simulink model "AttitudeControl_ADRC_FLY"  (R2017b)
settings: Solver=FixedStepDiscrete  StartTime=0.0  StopTime=10.0  RelTol=1e-3
undefined symbols (not defined in the file): DiscIntNeverNeededParam, Kd_YAW_AngleRate, Ki_YAW_AngleRate, Kp_YAW_AngleRate, RC1_MAX, RC1_MIN, RC2_MAX, RC2_MIN, RC3_MAX, RC3_MIN, RC4_MAX, RC4_MIN, RGBLED_COLOR_ENUM, RGBLED_MODE_ENUM, Saturation_I_Y_Max, Saturation_I_Y_Min, SL_ESO_B0, SL_ESO_B01, SL_ESO_B02, SL_ESO_B03, SL_ESO_D, SL_ESO_H, SL_NLSEF_C, SL_NLSEF_H, SL_NLSEF_R, SL_TD_H, SL_TD_R, tau2sigma, THR_HOVER
libraries: pixhawk_slib_sensors_actuators x5, simulink x2, pixhawk_slib_misc_utils x2
settings Model: Creator=wsh  LastModifiedBy=Mr Wang
settings OptimizationCC: DefaultParameterBehavior=Inlined  MaxStackSize=64
settings DebuggingCC: ParameterTunabilityLossMsg=error
settings HardwareCC: ProdBitPerPointer=32  ProdBitPerSizeT=32  ProdBitPerPtrDiffT=32  ProdLargestAtomicInteger=Long  ProdLargestAtomicFloat=Double  ProdWordSize=32  ProdHWDeviceType=ARM Compatible->ARM Cortex
settings SFSimCC: MATLABDynamicMemAlloc=off
settings RTWCC: SystemTargetFile=ert.tlc  HardwareBoard=Pixhawk PX4  TemplateMakefile=ert_default_tmf  GenerateReport=on  CustomSource=px4_simulink_app_params.c  Toolchain=Pixhawk Toolchain  IncludeHyperlinkInReport=on  LaunchReport=on  GenerateTraceInfo=on  GenerateTraceReport=on  GenerateTraceReportSl=on  GenerateTraceReportSf=on  GenerateTraceReportEml=on
settings CodeAppCC: ForceParamTrailComments=on  IgnoreCustomStorageClasses=off  OperatorAnnotations=on  SimulinkDataObjDesc=on  SFDataObjDesc=on  MATLABFcnDesc=on  InsertBlockDesc=on  StateflowObjectComments=on  MATLABSourceComments=on
settings ERTTargetCC: MultiwordLength=2048  ERTCustomFileTemplate=PX4_codertarget_file_process.tlc

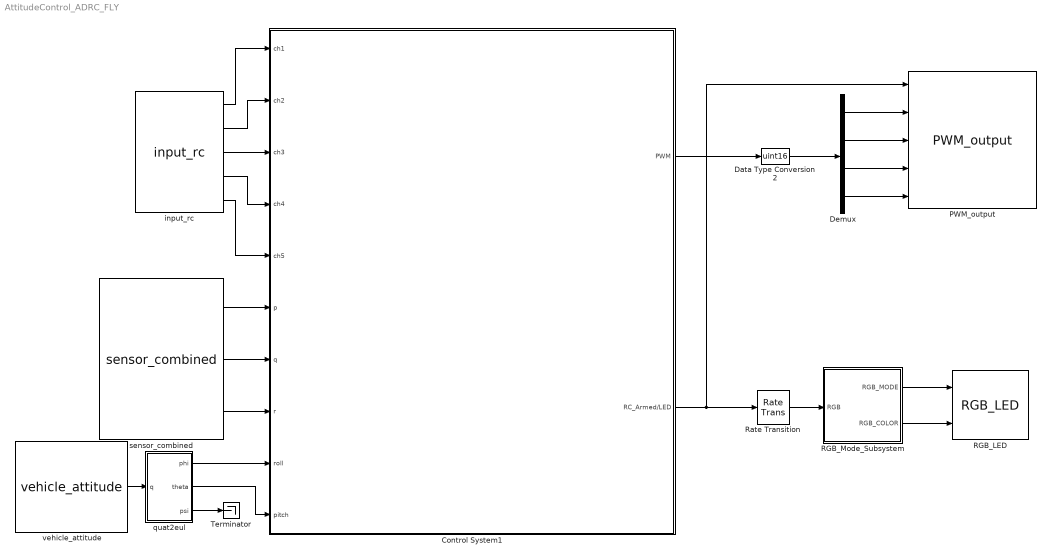
== system AttitudeControl_ADRC_FLY ==
  Control System1 : Subsystem
      mask Display: image('icon\pixhawk.png');
  Data Type Conversion2 : DataTypeConversion  OutDataTypeStr=uint16
  Demux : Demux
  PWM_output : pixhawk_slib_sensors_actuators/PWM_output  Description=|  pub_outputs=on  pwm_rate=400Hz  show_pwm1=on  show_pwm5=off  show_pwm2=on  show_pwm6=off  show_pwm3=on  show_pwm7=off  show_pwm4=on  show_pwm8=off
      | This block allows the user to send the appropriate PWM signals out to the PX4 outputs.  
      | These are usually connected to the ESCs which control the motor speeds. 
      | In order for the flight control to arm (enable) the output from the software side, the ARM Output input must be held high (boolean TRUE).  
      | Only then will the PWM values be sent out the PX4 hardware ports.  
      | This is usually a function of the RC Tx in combination with other flight modes programmed in the Simulink model by the user.  
      | The block has 8 available ports (data type uint16) which can be selectively chosen.  
      | These correspond to the 8 PWM output ports on the px4fmu hardware.
      settings: SourceProductName=Pixhawk Target Blocks
  RGB_LED : pixhawk_slib_sensors_actuators/RGB_LED
      settings: SourceProductName=Pixhawk Target Blocks
  RGB_Mode_Subsystem : Subsystem
  Rate Transition : RateTransition  OutPortSampleTime=1
  Terminator : Terminator
  input_rc : pixhawk_slib_sensors_actuators/input_rc  Description=|  sampletime=0.004  channel1=on  channel2=on  channel3=on  channel4=on  channel5=on  channel6=off  channel7=off  channel8=off  channel9=off  channel10=off  channel11=off  channel12=off  channel13=off  channel14=off  channel15=off  channel16=off  channel17=off  channel18=off  ch_count=off  rssi=off  rc_failsafe=off  rc_lost=off  rc_inputsource=off
      | RC Input Block
      | 
      | This block provides user input control to the model.
      | It uses the input_rc uORB topic.
      | 
      | The user has the ability to choose which channels are available as outputs from this block and also some optional outputs. These include 
      | Channels 1 through 18
      | double data type indicating the PWM value from the controller 
      | measured pulse widths for each of the supported channels 
      | Channel Count 
      | uint32 data type of the number of channels which are detector by the PX4 
      | RC Failsafe 
      | boolean data types indicating that the RC Tx is sending the FailSafe signal (if equipped and properly setup) 
      | explicit failsafe flag: true on TX failure or TX out of range , false otherwise. 
      | Only the true state is reliable, as there are some (PPM) receivers on the market going into failsafe without telling us explicitly. 
      | RC Input Source 
      | Enumeration data type indicating which source the RC input is from. 
      | Valid values are found in the ENUM file: RC_INPUT_SOURCE_ENUM.m 
      |           Enumeration members for class 'RC_INPUT_SOURCE_ENUM':
      |           RCINPUT_SOURCE_UNKNOWN         (0)
      |           RCINPUT_SOURCE_PX4FMU_PPM      (1)
      |           RCINPUT_SOURCE_PX4IO_PPM       (2)
      |           RCINPUT_SOURCE_PX4IO_SPEKTRUM  (3)
      |           RCINPUT_SOURCE_PX4IO_SBUS      (4)
      |           RCINPUT_SOURCE_PX4IO_ST24      (5)
      |           RCINPUT_SOURCE_MAVLINK         (6)
      |           RCINPUT_SOURCE_QURT            (7)
      |           RCINPUT_SOURCE_PX4FMU_SPEKTRUM (8)
      |           RCINPUT_SOURCE_PX4FMU_SBUS     (9)
      |           RCINPUT_SOURCE_PX4FMU_ST24     (10)
      |           RCINPUT_SOURCE_PX4FMU_SUMD     (11)
      |           RCINPUT_SOURCE_PX4FMU_DSM      (12)
      |           RCINPUT_SOURCE_PX4IO_SUMD      (13)
      | 
      | RSSI - Receive signal strength index 
      | receive signal strength indicator (RSSI): < 0: Undefined, 0: no signal, 255: full reception 
      | RC Lost Connection 
      | boolean data type indicating RC receiver connection status 
      | True, if no frame has arrived in the expected time, false otherwise. 
      | True usally means that the receiver has been disconnected, but can also indicate a radio link loss on "stupid" systems. 
      | Will remain false, if a RX with failsafe option continues to transmit frames after a link loss. 
      |   
      | Sample Model: px4demo_input_rc.slx
      settings: SourceProductName=Pixhawk Target Blocks
  quat2eul : MATLAB Function  TreatAsAtomicUnit=on
  sensor_combined : pixhawk_slib_sensors_actuators/sensor_combined  Description=|  sampletime=0.004  show_mag=off  show_acc=off  show_gyro=on  show_baro=off  show_ts=off
      | Sensor Combined Block
      | 
      | This block enables access to the various sensors available on the px4fmu-v2 hardware.  
      | The user can use these signals in the Simulink control model.  
      | The sample time needs to be provided in the mask dialog.  
      | Optional output ports can also be selected.  
      | Refer to the sample model: px4demo_attitude_control.slx
      | 
      | Signal definitions: 
      | Magnetometer (x,y,z) - single values – Magnetic field in NED body frame, in Gauss 
      | Accelerometer (x,y,z) - single values – Acceleration in NED body frame, in m/s^2 
      | Gyroscope (p,q,r) - single values – Angular velocity in radians per second 
      | Barometer (Altitude) - single value – Barometric pressure, already temperature compensated (millibars) 
      | RunTime (timestamp) - double value – Timestamp in microseconds since boot, from gyro 
      |   
      | The sensor_combined block needs to have the px4io service running on the PX4 hardware in order to get valid signal values.
      settings: SourceProductName=Pixhawk Target Blocks
  vehicle_attitude : pixhawk_slib_sensors_actuators/vehicle_attitude  Description=|  sampletime=0.004  show_r=off  show_p=off  show_y=off  show_q=on  show_ts=off
      | This block gives access to the running service that calculates the vehicle’s attitude.  A uORB topic (vehicle_attitude (attitude measurements)) publisher MUST be running in order for this block to provide valid signal values.  The available ones as of v1.3 are: 
      | attitude_estimator_ekf – EKF-Extended Kalman Filter for attitude estimation 
      | attitude_estimator_so3 – SO(3)-attitude estimation by using accelerometer, gyroscopes and magnetometer 
      | One of these MUST be running on the px4fmu in order for this block to return valid values.  Refer to the sample model: px4demo_attitude_control.slx. Attitude in NED (North-East-Down) body frame in SI units. 
      | Signal definitions: 
      | Roll – single value, Roll angle (rad, Tait-Bryan, NED) 
      | Pitch – single value, Pitch angle (rad, Tait-Bryan, NED) 
      | Yaw – single value, Yaw angle (rad, Tait-Bryan, NED) 
      | Quaternion (NED) – single(4) values (optional based on the uORB publisher)
      settings: SourceProductName=Pixhawk Target Blocks
  wires:
  sensor_combined/1 -> Control System1/6(p)
  sensor_combined/3 -> Control System1/8(r)
  sensor_combined/2 -> Control System1/7(q)
  input_rc/1 -> Control System1/1(ch1)
  input_rc/2 -> Control System1/2(ch2)
  input_rc/3 -> Control System1/3(ch3)
  input_rc/4 -> Control System1/4(ch4)
  input_rc/5 -> Control System1/5(ch5)
  quat2eul/2(theta) -> Control System1/10(pitch)
  quat2eul/3(psi) -> Terminator/1
  quat2eul/1(phi) -> Control System1/9(roll)
  vehicle_attitude/1 -> quat2eul/1(q)
  RGB_Mode_Subsystem/1(RGB_MODE) -> RGB_LED/1
  Rate Transition/1 -> RGB_Mode_Subsystem/1(RGB)
  RGB_Mode_Subsystem/2(RGB_COLOR) -> RGB_LED/2
  Control System1/2(RC_Armed/LED) -> PWM_output/1, Rate Transition/1
  Demux/3 -> PWM_output/4
  Data Type Conversion2/1 -> Demux/1
  Control System1/1(PWM) -> Data Type Conversion2/1
  Demux/4 -> PWM_output/5
  Demux/1 -> PWM_output/2
  Demux/2 -> PWM_output/3

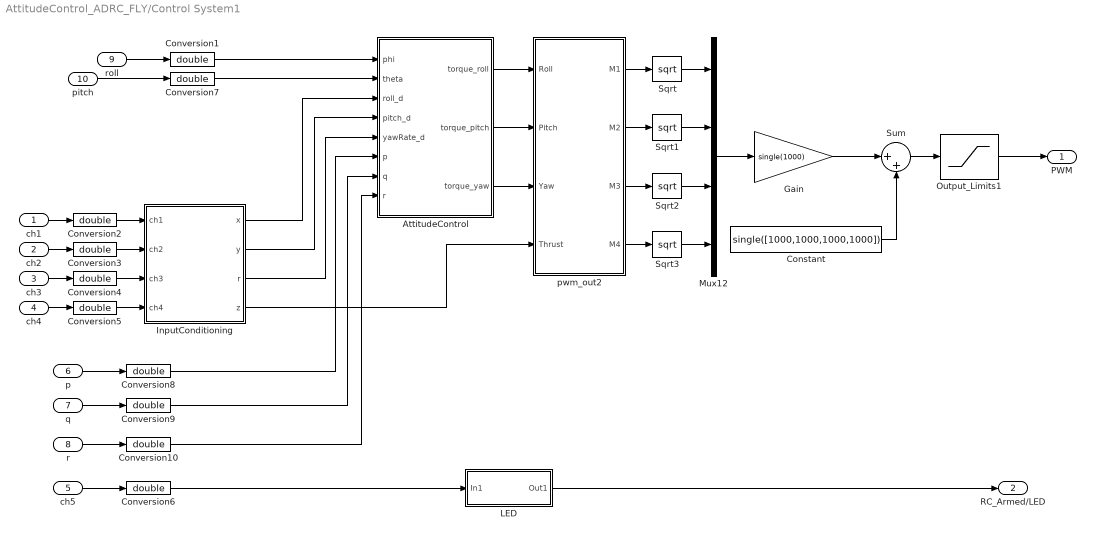
== system AttitudeControl_ADRC_FLY/Control System1 ==
  ch1 : Inport  OutDataTypeStr=uint16  PortDimensions=1
  ch2 : Inport  Port=2  OutDataTypeStr=uint16  PortDimensions=1
  ch3 : Inport  Port=3  OutDataTypeStr=uint16  PortDimensions=1
  ch4 : Inport  Port=4  OutDataTypeStr=uint16  PortDimensions=1
  ch5 : Inport  Port=5  OutDataTypeStr=uint16  PortDimensions=1  Interpolate=off
  p : Inport  Port=6  PortDimensions=1
  q : Inport  Port=7  PortDimensions=1
  r : Inport  Port=8  PortDimensions=1
  roll : Inport  Port=9  PortDimensions=1
  pitch : Inport  Port=10  PortDimensions=1
  AttitudeControl : Subsystem
  Constant : Constant  Value=single([1000,1000,1000,1000])
  Conversion{1..10} (10 alike) : DataTypeConversion  OutDataTypeStr=double
  Gain : Gain  Gain=single(1000)
  InputConditioning : Subsystem
  "LED " : Subsystem
  Mux12 : Mux
  Output_Limits1 : Saturate  Priority=2  UpperLimit=2000  LowerLimit=1000
  Sqrt{,1..3} (4 alike) : Sqrt  SaturateOnIntegerOverflow=on
  Sum : Sum  Inputs=|++
  pwm_out2 : MATLAB Function  SystemSampleTime=0.004
  PWM : Outport
  RC_Armed/LED : Outport  Port=2  PortDimensions=1
  wires:
  ch3/1 -> Conversion4/1
  ch5/1 -> Conversion6/1
  r/1 -> Conversion10/1
  q/1 -> Conversion9/1
  InputConditioning/3(r) -> AttitudeControl/5(yawRate_d)
  p/1 -> Conversion8/1
  ch4/1 -> Conversion5/1
  "LED "/1(Out1) -> RC_Armed/LED/1
  Conversion6/1 -> "LED "/1(In1)
  Conversion5/1 -> InputConditioning/4(ch4)
  Conversion4/1 -> InputConditioning/3(ch3)
  pitch/1 -> Conversion7/1
  roll/1 -> Conversion1/1
  ch1/1 -> Conversion2/1
  ch2/1 -> Conversion3/1
  Conversion1/1 -> AttitudeControl/1(phi)
  Conversion7/1 -> AttitudeControl/2(theta)
  Conversion8/1 -> AttitudeControl/6(p)
  Conversion9/1 -> AttitudeControl/7(q)
  Conversion10/1 -> AttitudeControl/8(r)
  Conversion2/1 -> InputConditioning/1("ch1 ")
  Conversion3/1 -> InputConditioning/2(ch2)
  InputConditioning/1(x) -> AttitudeControl/3(roll_d)
  InputConditioning/2(y) -> AttitudeControl/4(pitch_d)
  Constant/1 -> Sum/2
  Gain/1 -> Sum/1
  Mux12/1 -> Gain/1
  Sqrt3/1 -> Mux12/4
  Sqrt1/1 -> Mux12/2
  Sqrt/1 -> Mux12/1
  InputConditioning/4(z) -> pwm_out2/4(Thrust)
  pwm_out2/1(M1) -> Sqrt/1
  pwm_out2/2(M2) -> Sqrt1/1
  AttitudeControl/2(torque_pitch) -> pwm_out2/2(Pitch)
  AttitudeControl/1(torque_roll) -> pwm_out2/1(Roll)
  Sum/1 -> Output_Limits1/1
  Sqrt2/1 -> Mux12/3
  AttitudeControl/3(torque_yaw) -> pwm_out2/3(Yaw)
  pwm_out2/3(M3) -> Sqrt2/1
  pwm_out2/4(M4) -> Sqrt3/1
  Output_Limits1/1 -> PWM/1

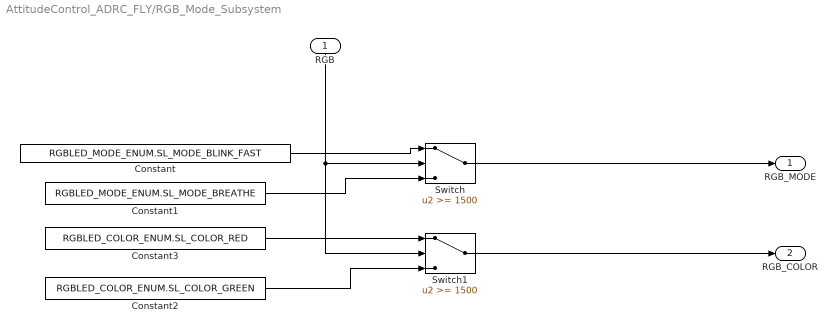
== system AttitudeControl_ADRC_FLY/RGB_Mode_Subsystem ==
  RGB : Inport
  Constant : Constant  Value=RGBLED_MODE_ENUM.SL_MODE_BLINK_FAST  OutDataTypeStr=Enum: RGBLED_MODE_ENUM
  Constant1 : Constant  Value=RGBLED_MODE_ENUM.SL_MODE_BREATHE  OutDataTypeStr=Enum: RGBLED_MODE_ENUM
  Constant2 : Constant  Value=RGBLED_COLOR_ENUM.SL_COLOR_GREEN  OutDataTypeStr=Enum: RGBLED_COLOR_ENUM
  Constant3 : Constant  Value=RGBLED_COLOR_ENUM.SL_COLOR_RED  OutDataTypeStr=Enum: RGBLED_COLOR_ENUM
  Switch : Switch  Threshold=1500
  Switch1 : Switch  Threshold=1500
  RGB_MODE : Outport
  RGB_COLOR : Outport  Port=2
  wires:
  Switch1/1 -> RGB_COLOR/1
  Constant2/1 -> Switch1/3
  Constant3/1 -> Switch1/1
  Switch/1 -> RGB_MODE/1
  Constant1/1 -> Switch/3
  Constant/1 -> Switch/1
  RGB/1 -> Switch/2, Switch1/2

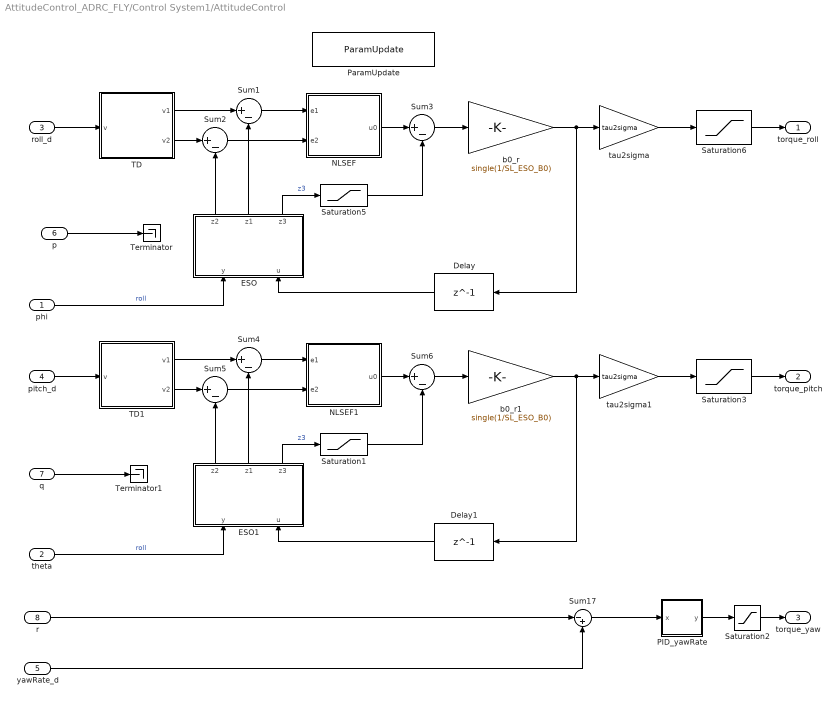
== system AttitudeControl_ADRC_FLY/Control System1/AttitudeControl ==
  phi : Inport
  theta : Inport  Port=2
  roll_d : Inport  Port=3
  pitch_d : Inport  Port=4
  yawRate_d : Inport  Port=5
  p : Inport  Port=6
  q : Inport  Port=7
  r : Inport  Port=8
  Delay : Delay  DelayLength=1  InitialCondition=0
  Delay1 : Delay  DelayLength=1  InitialCondition=0
  ESO : Subsystem
  ESO1 : Subsystem
  NLSEF : Subsystem
  NLSEF1 : Subsystem
  PID_yawRate : Subsystem
  ParamUpdate : pixhawk_slib_misc_utils/ParamUpdate  Description=|  Unformatted_StrSet=0  TLC_StrSet=0  NumParams=0  Ts=0
      | ParamUpdate Block
      | 
      | Use this block at your top-level of your model to insert a "parameter update" function in the generated code.
      settings: SourceProductName=Pixhawk Target Blocks
  Saturation1 : Saturate  UpperLimit=SL_NLSEF_R*0.5  LowerLimit=-SL_NLSEF_R*0.5
  Saturation2 : Saturate
  Saturation3 : Saturate  UpperLimit=0.4  LowerLimit=-0.4
  Saturation5 : Saturate  UpperLimit=SL_NLSEF_R*0.5  LowerLimit=-SL_NLSEF_R*0.5
  Saturation6 : Saturate  UpperLimit=0.4  LowerLimit=-0.4
  Sum{1..6} (6 alike) : Sum  Inputs=|+-
  Sum17 : Sum  Inputs=|-+
  TD : Subsystem
  TD1 : Subsystem
  Terminator : Terminator
  Terminator1 : Terminator
  b0_r : Gain  Gain=single(1/SL_ESO_B0)
  b0_r1 : Gain  Gain=single(1/SL_ESO_B0)
  tau2sigma : Gain  Gain=tau2sigma
  tau2sigma1 : Gain  Gain=tau2sigma
  torque_roll : Outport
  torque_pitch : Outport  Port=2
  torque_yaw : Outport  Port=3
  wires:
  r/1 -> Sum17/1
  Sum17/1 -> PID_yawRate/1(x)
  PID_yawRate/1(y) -> Saturation2/1
  yawRate_d/1 -> Sum17/2
  Saturation2/1 -> torque_yaw/1
  ESO/1(z2) -> Sum2/2
  ESO/3(z3) -> Saturation5/1  "z3"
  roll_d/1 -> TD/1(v)
  ESO/2(z1) -> Sum1/2
  Saturation5/1 -> Sum3/2
  Sum3/1 -> b0_r/1
  TD/1(v1) -> Sum1/1
  Delay/1 -> ESO/2(u)
  tau2sigma/1 -> Saturation6/1
  b0_r/1 -> tau2sigma/1, Delay/1
  Sum1/1 -> NLSEF/1(e1)
  phi/1 -> ESO/1(y)  "roll"
  NLSEF/1(u0) -> Sum3/1
  Saturation6/1 -> torque_roll/1
  TD/2(v2) -> Sum2/1
  Sum2/1 -> NLSEF/2(e2)
  theta/1 -> ESO1/1(y)  "roll"
  pitch_d/1 -> TD1/1(v)
  Sum5/1 -> NLSEF1/2(e2)
  TD1/2(v2) -> Sum5/1
  NLSEF1/1(u0) -> Sum6/1
  Delay1/1 -> ESO1/2(u)
  Saturation3/1 -> torque_pitch/1
  b0_r1/1 -> tau2sigma1/1, Delay1/1
  TD1/1(v1) -> Sum4/1
  tau2sigma1/1 -> Saturation3/1
  Sum4/1 -> NLSEF1/1(e1)
  ESO1/3(z3) -> Saturation1/1  "z3"
  Saturation1/1 -> Sum6/2
  ESO1/2(z1) -> Sum4/2
  ESO1/1(z2) -> Sum5/2
  Sum6/1 -> b0_r1/1
  p/1 -> Terminator/1
  q/1 -> Terminator1/1

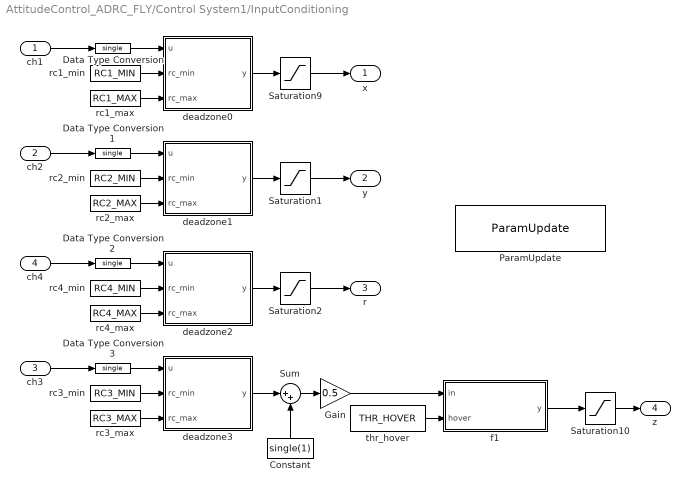
== system AttitudeControl_ADRC_FLY/Control System1/InputConditioning ==
  "ch1 " : Inport
  ch2 : Inport  Port=2
  ch3 : Inport  Port=3
  ch4 : Inport  Port=4
  Constant : Constant  Value=single(1)
  Data Type Conversion{,1..3} (4 alike) : DataTypeConversion  OutDataTypeStr=single
  Gain : Gain  Gain=0.5  ParamDataTypeStr=single  OutDataTypeStr=single
  ParamUpdate : pixhawk_slib_misc_utils/ParamUpdate  Description=|  Unformatted_StrSet=0  TLC_StrSet=0  NumParams=0  Ts=0
      | ParamUpdate Block
      | 
      | Use this block at your top-level of your model to insert a "parameter update" function in the generated code.
      settings: SourceProductName=Pixhawk Target Blocks
  Saturation1 : Saturate  UpperLimit=1  LowerLimit=-1
  Saturation10 : Saturate  UpperLimit=1  LowerLimit=0
  Saturation2 : Saturate  UpperLimit=1  LowerLimit=-1
  Saturation9 : Saturate  UpperLimit=1  LowerLimit=-1
  Sum : Sum  Inputs=|++
  deadzone0 : MATLAB Function  TreatAsAtomicUnit=on
  deadzone1 : MATLAB Function  TreatAsAtomicUnit=on
  deadzone2 : MATLAB Function  TreatAsAtomicUnit=on
  deadzone3 : MATLAB Function  TreatAsAtomicUnit=on
  f1 : MATLAB Function  TreatAsAtomicUnit=on
  rc1_max : Constant  Value=RC1_MAX
  rc1_min : Constant  Value=RC1_MIN
  rc2_max : Constant  Value=RC2_MAX
  rc2_min : Constant  Value=RC2_MIN
  rc3_max : Constant  Value=RC3_MAX
  rc3_min : Constant  Value=RC3_MIN
  rc4_max : Constant  Value=RC4_MAX
  rc4_min : Constant  Value=RC4_MIN
  "thr_hover " : Constant  Value=THR_HOVER  OutDataTypeStr=single
  x : Outport
  y : Outport  Port=2
  r : Outport  Port=3
  z : Outport  Port=4
  wires:
  f1/1(y) -> Saturation10/1
  Gain/1 -> f1/1(in)
  "thr_hover "/1 -> f1/2(hover)
  Sum/1 -> Gain/1
  Constant/1 -> Sum/2
  "ch1 "/1 -> Data Type Conversion/1
  deadzone0/1(y) -> Saturation9/1
  Saturation10/1 -> z/1
  deadzone3/1(y) -> Sum/1
  rc1_min/1 -> deadzone0/2(rc_min)
  rc1_max/1 -> deadzone0/3(rc_max)
  Data Type Conversion/1 -> deadzone0/1(u)
  Data Type Conversion1/1 -> deadzone1/1(u)
  rc2_max/1 -> deadzone1/3(rc_max)
  rc2_min/1 -> deadzone1/2(rc_min)
  deadzone1/1(y) -> Saturation1/1
  ch2/1 -> Data Type Conversion1/1
  Data Type Conversion2/1 -> deadzone2/1(u)
  rc4_max/1 -> deadzone2/3(rc_max)
  rc4_min/1 -> deadzone2/2(rc_min)
  deadzone2/1(y) -> Saturation2/1
  ch4/1 -> Data Type Conversion2/1
  Saturation2/1 -> r/1
  ch3/1 -> Data Type Conversion3/1
  rc3_min/1 -> deadzone3/2(rc_min)
  rc3_max/1 -> deadzone3/3(rc_max)
  Data Type Conversion3/1 -> deadzone3/1(u)
  Saturation9/1 -> x/1
  Saturation1/1 -> y/1

== system AttitudeControl_ADRC_FLY/Control System1/LED  ==
  In1 : Inport
  Compare To Constant3 : simulink/Logic and Bit Operations/Compare To Constant  relop=>=  const=uint16(1500)  OutDataTypeStr=boolean
  Out1 : Outport
  wires:
  Compare To Constant3/1 -> Out1/1
  In1/1 -> Compare To Constant3/1

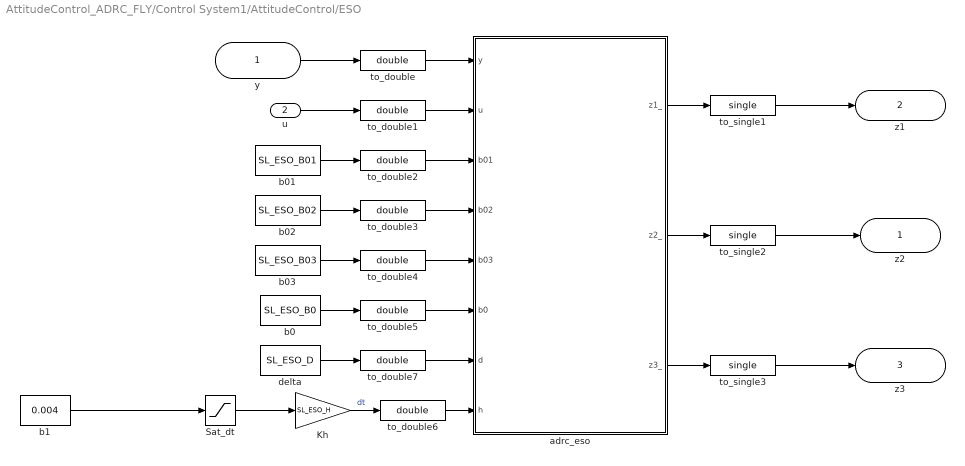
== system AttitudeControl_ADRC_FLY/Control System1/AttitudeControl/ESO ==
  y : Inport
  u : Inport  Port=2
  Kh : Gain  Priority=4  Gain=SL_ESO_H
  Sat_dt : Saturate  UpperLimit=0.02  LowerLimit=0.004
  adrc_eso : MATLAB Function  TreatAsAtomicUnit=on
  b0 : Constant  Value=SL_ESO_B0
  b01 : Constant  Value=SL_ESO_B01
  b02 : Constant  Value=SL_ESO_B02
  b03 : Constant  Value=SL_ESO_B03
  b1 : Constant  Value=0.004
  delta : Constant  Value=SL_ESO_D
  to_double{,1..7} (8 alike) : DataTypeConversion  OutDataTypeStr=double
  to_single1 : DataTypeConversion  OutDataTypeStr=single
  to_single2 : DataTypeConversion  OutDataTypeStr=single
  to_single3 : DataTypeConversion  OutDataTypeStr=single
  z2 : Outport
  z1 : Outport  Port=2  OutDataTypeStr=single
  z3 : Outport  Port=3
  wires:
  y/1 -> to_double/1
  u/1 -> to_double1/1
  b1/1 -> Sat_dt/1
  Sat_dt/1 -> Kh/1
  Kh/1 -> to_double6/1  "dt"
  adrc_eso/1(z1_) -> to_single1/1
  adrc_eso/2(z2_) -> to_single2/1
  adrc_eso/3(z3_) -> to_single3/1
  b01/1 -> to_double2/1
  b02/1 -> to_double3/1
  b03/1 -> to_double4/1
  b0/1 -> to_double5/1
  to_double/1 -> adrc_eso/1(y)
  to_double1/1 -> adrc_eso/2(u)
  to_double2/1 -> adrc_eso/3(b01)
  to_double3/1 -> adrc_eso/4(b02)
  to_double4/1 -> adrc_eso/5(b03)
  to_double5/1 -> adrc_eso/6(b0)
  to_single1/1 -> z1/1
  to_single2/1 -> z2/1
  to_single3/1 -> z3/1
  to_double6/1 -> adrc_eso/8(h)
  delta/1 -> to_double7/1
  to_double7/1 -> adrc_eso/7(d)

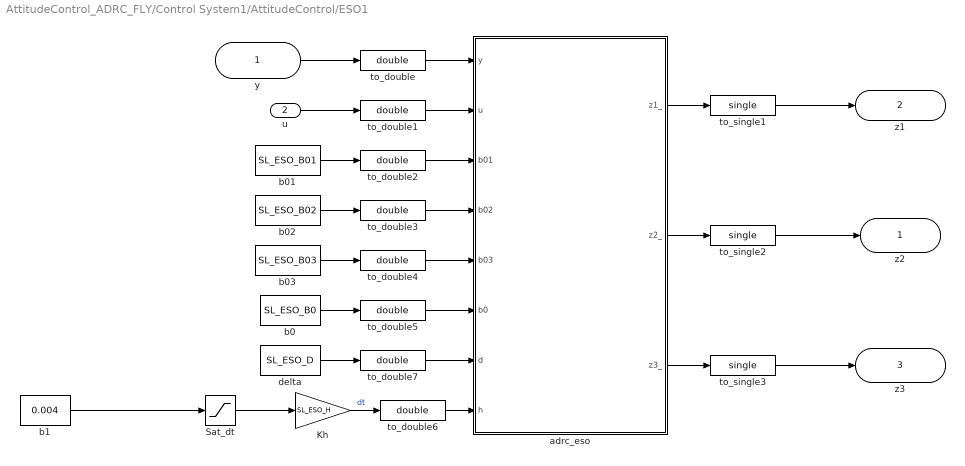
== system AttitudeControl_ADRC_FLY/Control System1/AttitudeControl/ESO1 ==
  y : Inport
  u : Inport  Port=2
  Kh : Gain  Priority=4  Gain=SL_ESO_H
  Sat_dt : Saturate  UpperLimit=0.02  LowerLimit=0.004
  adrc_eso : MATLAB Function  TreatAsAtomicUnit=on
  b0 : Constant  Value=SL_ESO_B0
  b01 : Constant  Value=SL_ESO_B01
  b02 : Constant  Value=SL_ESO_B02
  b03 : Constant  Value=SL_ESO_B03
  b1 : Constant  Value=0.004
  delta : Constant  Value=SL_ESO_D
  to_double{,1..7} (8 alike) : DataTypeConversion  OutDataTypeStr=double
  to_single1 : DataTypeConversion  OutDataTypeStr=single
  to_single2 : DataTypeConversion  OutDataTypeStr=single
  to_single3 : DataTypeConversion  OutDataTypeStr=single
  z2 : Outport
  z1 : Outport  Port=2  OutDataTypeStr=single
  z3 : Outport  Port=3
  wires:
  to_double7/1 -> adrc_eso/7(d)
  delta/1 -> to_double7/1
  to_double6/1 -> adrc_eso/8(h)
  to_single3/1 -> z3/1
  to_single2/1 -> z2/1
  to_single1/1 -> z1/1
  to_double5/1 -> adrc_eso/6(b0)
  to_double4/1 -> adrc_eso/5(b03)
  to_double3/1 -> adrc_eso/4(b02)
  to_double2/1 -> adrc_eso/3(b01)
  to_double1/1 -> adrc_eso/2(u)
  to_double/1 -> adrc_eso/1(y)
  b0/1 -> to_double5/1
  b03/1 -> to_double4/1
  b02/1 -> to_double3/1
  b01/1 -> to_double2/1
  adrc_eso/3(z3_) -> to_single3/1
  adrc_eso/2(z2_) -> to_single2/1
  adrc_eso/1(z1_) -> to_single1/1
  Kh/1 -> to_double6/1  "dt"
  Sat_dt/1 -> Kh/1
  b1/1 -> Sat_dt/1
  u/1 -> to_double1/1
  y/1 -> to_double/1

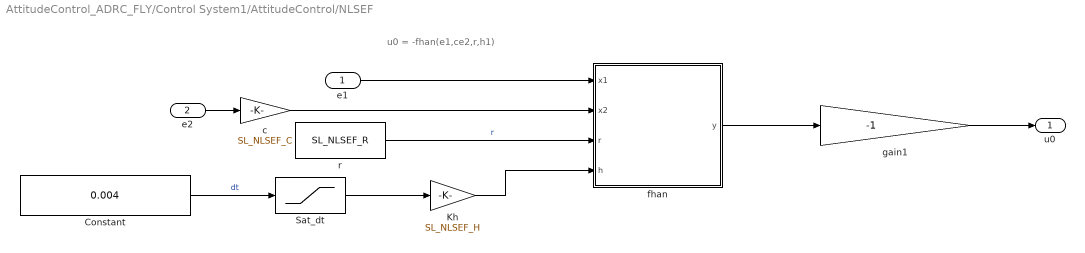
== system AttitudeControl_ADRC_FLY/Control System1/AttitudeControl/NLSEF ==
  note: u0 = -fhan(e1,ce2,r,h1)
  e1 : Inport
  e2 : Inport  Port=2
  Constant : Constant  Value=0.004  OutDataTypeStr=single
  Kh : Gain  Gain=SL_NLSEF_H
  Sat_dt : Saturate  UpperLimit=0.02  LowerLimit=0.004
  c : Gain  Gain=SL_NLSEF_C
  fhan : MATLAB Function  TreatAsAtomicUnit=on
  gain1 : Gain  Gain=-1
  r : Constant  Value=SL_NLSEF_R
  u0 : Outport
  wires:
  Kh/1 -> fhan/4(h)
  gain1/1 -> u0/1
  e1/1 -> fhan/1(x1)
  e2/1 -> c/1
  r/1 -> fhan/3(r)  "r"
  c/1 -> fhan/2(x2)
  Sat_dt/1 -> Kh/1
  fhan/1(y) -> gain1/1
  Constant/1 -> Sat_dt/1  "dt"

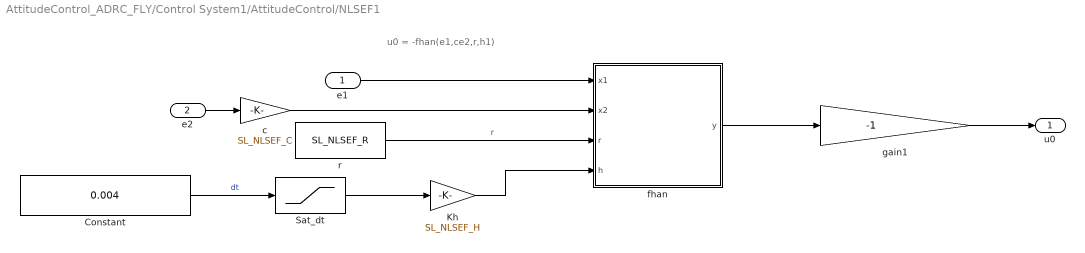
== system AttitudeControl_ADRC_FLY/Control System1/AttitudeControl/NLSEF1 ==
  note: u0 = -fhan(e1,ce2,r,h1)
  e1 : Inport
  e2 : Inport  Port=2
  Constant : Constant  Value=0.004  OutDataTypeStr=single
  Kh : Gain  Gain=SL_NLSEF_H
  Sat_dt : Saturate  UpperLimit=0.02  LowerLimit=0.004
  c : Gain  Gain=SL_NLSEF_C
  fhan : MATLAB Function  TreatAsAtomicUnit=on
  gain1 : Gain  Gain=-1
  r : Constant  Value=SL_NLSEF_R
  u0 : Outport
  wires:
  Constant/1 -> Sat_dt/1  "dt"
  fhan/1(y) -> gain1/1
  Sat_dt/1 -> Kh/1
  c/1 -> fhan/2(x2)
  r/1 -> fhan/3(r)  "r"
  e2/1 -> c/1
  e1/1 -> fhan/1(x1)
  gain1/1 -> u0/1
  Kh/1 -> fhan/4(h)

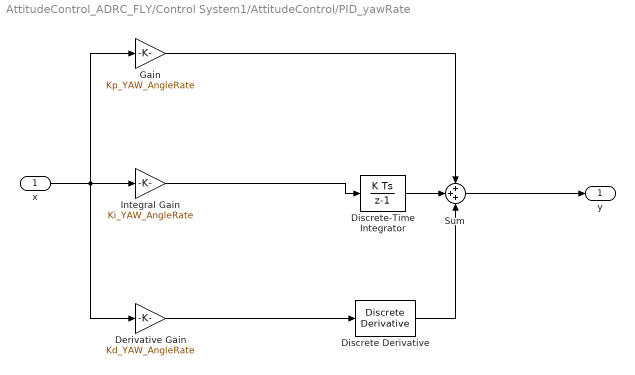
== system AttitudeControl_ADRC_FLY/Control System1/AttitudeControl/PID_yawRate ==
  x : Inport
  Derivative Gain : Gain  DisableCoverage=on  Gain=Kd_YAW_AngleRate  ParamMin=-100  ParamMax=100  OutMin=-100  OutMax=100
  Discrete Derivative : simulink/Discrete/Discrete Derivative  gainval=1.0  ICPrevScaledInput=0.0  OutMin=[]  OutMax=[]  OutDataType=fixdt(1, 16)  OutScaling=2^-10  DoSatur=off
  Discrete-Time Integrator : DiscreteIntegrator  InitialConditionSetting=State (most efficient)  SampleTime=-1  LimitOutput=on  UpperSaturationLimit=Saturation_I_Y_Max  LowerSaturationLimit=Saturation_I_Y_Min  ICPrevOutput=DiscIntNeverNeededParam  ICPrevScaledInput=DiscIntNeverNeededParam
  Gain : Gain  Gain=Kp_YAW_AngleRate
  Integral Gain : Gain  DisableCoverage=on  Gain=Ki_YAW_AngleRate
  Sum : Sum  Inputs=+++
  y : Outport  InitialOutput=0
  wires:
  x/1 -> Gain/1, Integral Gain/1, Derivative Gain/1
  Integral Gain/1 -> Discrete-Time Integrator/1
  Derivative Gain/1 -> Discrete Derivative/1
  Gain/1 -> Sum/1
  Sum/1 -> y/1
  Discrete Derivative/1 -> Sum/3
  Discrete-Time Integrator/1 -> Sum/2

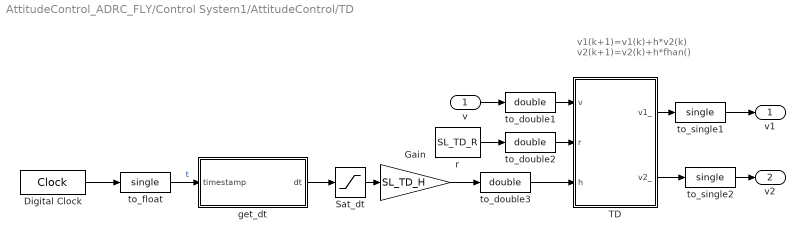
== system AttitudeControl_ADRC_FLY/Control System1/AttitudeControl/TD ==
  note: v1(k+1)=v1(k)+h*v2(k)
      | v2(k+1)=v2(k)+h*fhan()
  v : Inport
  Digital Clock : DigitalClock  SampleTime=-1
  Gain : Gain  Gain=SL_TD_H
  Sat_dt : Saturate  UpperLimit=0.02  LowerLimit=0.004
  TD : MATLAB Function  TreatAsAtomicUnit=on
  get_dt : MATLAB Function  TreatAsAtomicUnit=on
  r : Constant  Value=SL_TD_R
  to_double1 : DataTypeConversion  OutDataTypeStr=double
  to_double2 : DataTypeConversion  OutDataTypeStr=double
  to_double3 : DataTypeConversion  OutDataTypeStr=double
  to_float : DataTypeConversion  OutDataTypeStr=single
  to_single1 : DataTypeConversion  OutDataTypeStr=single
  to_single2 : DataTypeConversion  OutDataTypeStr=single
  v1 : Outport
  v2 : Outport  Port=2
  wires:
  v/1 -> to_double1/1
  TD/1(v1_) -> to_single1/1
  r/1 -> to_double2/1
  TD/2(v2_) -> to_single2/1
  get_dt/1(dt) -> Sat_dt/1
  to_float/1 -> get_dt/1(timestamp)  "t"
  Sat_dt/1 -> Gain/1
  Digital Clock/1 -> to_float/1
  Gain/1 -> to_double3/1
  to_double1/1 -> TD/1(v)
  to_double2/1 -> TD/2(r)
  to_double3/1 -> TD/3(h)
  to_single1/1 -> v1/1
  to_single2/1 -> v2/1

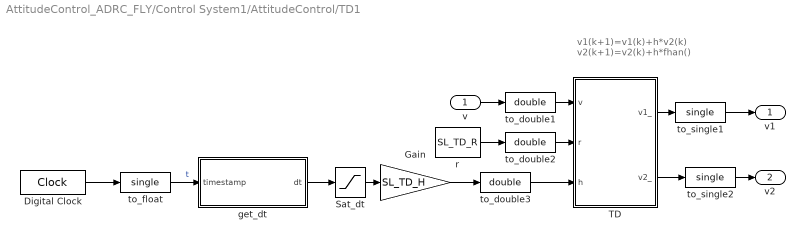
== system AttitudeControl_ADRC_FLY/Control System1/AttitudeControl/TD1 ==
  note: v1(k+1)=v1(k)+h*v2(k)
      | v2(k+1)=v2(k)+h*fhan()
  v : Inport
  Digital Clock : DigitalClock  SampleTime=-1
  Gain : Gain  Gain=SL_TD_H
  Sat_dt : Saturate  UpperLimit=0.02  LowerLimit=0.004
  TD : MATLAB Function  TreatAsAtomicUnit=on
  get_dt : MATLAB Function  TreatAsAtomicUnit=on
  r : Constant  Value=SL_TD_R
  to_double1 : DataTypeConversion  OutDataTypeStr=double
  to_double2 : DataTypeConversion  OutDataTypeStr=double
  to_double3 : DataTypeConversion  OutDataTypeStr=double
  to_float : DataTypeConversion  OutDataTypeStr=single
  to_single1 : DataTypeConversion  OutDataTypeStr=single
  to_single2 : DataTypeConversion  OutDataTypeStr=single
  v1 : Outport
  v2 : Outport  Port=2
  wires:
  to_single2/1 -> v2/1
  to_single1/1 -> v1/1
  to_double3/1 -> TD/3(h)
  to_double2/1 -> TD/2(r)
  to_double1/1 -> TD/1(v)
  Gain/1 -> to_double3/1
  Digital Clock/1 -> to_float/1
  Sat_dt/1 -> Gain/1
  to_float/1 -> get_dt/1(timestamp)  "t"
  get_dt/1(dt) -> Sat_dt/1
  TD/2(v2_) -> to_single2/1
  r/1 -> to_double2/1
  TD/1(v1_) -> to_single1/1
  v/1 -> to_double1/1

== matlab function AttitudeControl_ADRC_FLY/Control System1/InputConditioning/deadzone0 ==
  data: u input; y output; rc_min input; rc_max input
function y = fcn(u, rc_min, rc_max)
%Function description:
%  Control the range of the remote control input from RCMin to RCMax, and set
%  a dead zone with a dead zone size of ±deadZone,the output y is
%  normalized to 0~1.You can get the RC calibration parameters in QGC.
RCMin = rc_min;
RCMax = rc_max;
RCMid = ((RCMin + RCMax)/2);
deadZoneRate = double(0.05);
deadZone = deadZoneRate*(RCMax - RCMin);
k = 1/(RCMax - RCMid - deadZone);
%Limiting
if(u < RCMin)
    u = RCMin;
elseif(u > RCMax)
    u = RCMax;
end
%dead zone and normalize
 if(u > RCMid + deadZone)
    y = single((u-RCMid - deadZone)*k);
 elseif(u < RCMid - deadZone)
     y = single((u - RCMid + deadZone)*k);
 else
     y = single(0);
 end
 end

== matlab function AttitudeControl_ADRC_FLY/Control System1/InputConditioning/deadzone1 ==
  data: u input; y output; rc_min input; rc_max input
function y = fcn(u, rc_min, rc_max)
%Function description:
%  Control the range of the remote control input from RCMin to RCMax, and set
%  a dead zone with a dead zone size of ±deadZone,the output y is
%  normalized to 0~1.You can get the RC calibration parameters in QGC.
RCMin = rc_min;
RCMax = rc_max;
RCMid = ((RCMin + RCMax)/2);
deadZoneRate = double(0.05);
deadZone = deadZoneRate*(RCMax - RCMin);
k = 1/(RCMax - RCMid - deadZone);
%Limiting
if(u < RCMin)
    u = RCMin;
elseif(u > RCMax)
    u = RCMax;
end
%dead zone and normalize
 if(u > RCMid + deadZone)
    y = single((u-RCMid - deadZone)*k);
 elseif(u < RCMid - deadZone)
     y = single((u - RCMid + deadZone)*k);
 else
     y = single(0);
 end
 end

== matlab function AttitudeControl_ADRC_FLY/Control System1/InputConditioning/deadzone3 ==
  data: u input; y output; rc_min input; rc_max input
function y = fcn(u, rc_min, rc_max)
%Function description:
%  Control the range of the remote control input from RCMin to RCMax, and set
%  a dead zone with a dead zone size of ±deadZone,the output y is
%  normalized to 0~1.You can get the RC calibration parameters in QGC.
RCMin = rc_min;
RCMax = rc_max;
RCMid = ((RCMin + RCMax)/2);
deadZoneRate = double(0.05);
deadZone = deadZoneRate*(RCMax - RCMin);
k = 1/(RCMax - RCMid - deadZone);
%Limiting
if(u < RCMin)
    u = RCMin;
elseif(u > RCMax)
    u = RCMax;
end
%dead zone and normalize
 if(u > RCMid + deadZone)
    y = single((u-RCMid - deadZone)*k);
 elseif(u < RCMid - deadZone)
     y = single((u - RCMid + deadZone)*k);
 else
     y = single(0);
 end
 end

== matlab function AttitudeControl_ADRC_FLY/Control System1/AttitudeControl/TD1/TD ==
  data: v input; v1_ output; r input; h input; v2_ output
function [v1_, v2_] = TD(v, r, h)
persistent v1 v2
if isempty(v1) || isempty(v2)
    v1 = 0;
    v2 = 0;
end

fv = fhan(v1 - v, v2, r,  h);
v1_ = v1 + h*v2;
v2_ = v2 + h*fv;

v1 = v1_;
v2 = v2_;
end

function y = fhan(x1, x2, r0, h0)

d = r0*h0^2;
a0 = h0*x2;
y = x1 + a0;
a1 = sqrt(d*(d + 8*abs(y)));
a2 = a0 + sign(y)*(a1 - d)/2;
sy = (sign(y + d) - sign(y - d))/2;%fsg
a = (a0 + y -a2)*sy + a2;
sa = (sign(a + d) - sign(a - d))/2;
y = -r0*(a/d - sign(a))*sa - r0*sign(a);

end

== matlab function AttitudeControl_ADRC_FLY/Control System1/InputConditioning/deadzone2 ==
  data: u input; y output; rc_min input; rc_max input
function y = fcn(u, rc_min, rc_max)
%Function description:
%  Control the range of the remote control input from RCMin to RCMax, and set
%  a dead zone with a dead zone size of ±deadZone,the output y is
%  normalized to 0~1.You can get the RC calibration parameters in QGC.
RCMin = rc_min;
RCMax = rc_max;
RCMid = ((RCMin + RCMax)/2);
deadZoneRate = double(0.05);
deadZone = deadZoneRate*(RCMax - RCMin);
k = 1/(RCMax - RCMid - deadZone);
%Limiting
if(u < RCMin)
    u = RCMin;
elseif(u > RCMax)
    u = RCMax;
end
%dead zone and normalize
 if(u > RCMid + deadZone)
    y = single((u-RCMid - deadZone)*k);
 elseif(u < RCMid - deadZone)
     y = single((u - RCMid + deadZone)*k);
 else
     y = single(0);
 end
 end

== matlab function AttitudeControl_ADRC_FLY/Control System1/AttitudeControl/TD1/get_dt ==
  data: timestamp input; dt output
function dt = get_dt(timestamp)
%timestamp: s
%dt :s
persistent t_last
if isempty(t_last)
    t_last = timestamp;
end
dt = timestamp - t_last;
t_last = timestamp;

== matlab function AttitudeControl_ADRC_FLY/Control System1/AttitudeControl/NLSEF1/fhan ==
  data: x1 input single; y output single; x2 input single; r input single; h input single
function y = fhan(x1, x2, r, h)
    d = r * h^2;
    a0 = h * x2;
    y = x1 + a0;
    a1 = sqrt( d * (d + 8*abs(y)) );
    a2 = a0 + sign(y)*(a1 - d)/2;
    sy = (sign(y + d) - sign(y - d))/2;
    a = (a0 + y - a2)*sy + a2;
    sa = (sign(a + d) - sign(a - d))/2;
    y = -r*(a/d - sign(a))*sa - r*sign(a);

== matlab function AttitudeControl_ADRC_FLY/Control System1/AttitudeControl/ESO1/adrc_eso ==
  data: y input; u input; z1_ output; b01 input; b02 input; b03 input; b0 input; d input; h input; z2_ output; z3_ output
function [z1_, z2_, z3_] = adrc_eso(y, u, b01, b02, b03, b0, d, h)
persistent z1  z2 z3
if (isempty(z1) || isempty(z2) || isempty(z3))
    z1 = 0;
    z2 = 0;
    z3 = 0;
end
e = z1 - y;
fe = fal(e, 0.5, d);
fe1 = fal(e, 0.25, d);

z1_ = z1 + h*(z2 - b01*e);
z2_ = z2 + h*(z3 + b0*u - b02*fe);
z3_ = z3 - h*b03*fe1;

z1 = z1_;
z2 = z2_;
z3 = z3_;

end

function  y = fal( x, alpha, delta )

if abs(x) < delta
    y = x / delta^(1.0 - alpha);
else
    y = (abs(x)^alpha) * sign(x);
end

end

== matlab function AttitudeControl_ADRC_FLY/quat2eul ==
  data: q input; phi output; theta output; psi output
function [phi,theta,psi] = quat2eul(q)
% Conversion from Quaternion to Euler angles based on the PX4 Firmware
% v1.6.5 release.
% 
% Quaternion -> DCM -> Euler Angles
% INPUT:
%   q: Quaternion vector of the format: (a + bi + cj + dk)
% OUTPUT:
%   [phi,theta,psi]: Euler angles in radians.
% 
 
    a = q(1);
    b = q(2);
    c = q(3);
    d = q(4);

    aSq = a*a;
    bSq = b*b;
    cSq = c*c;
    dSq = d*d;

    d_pi2 = pi/2;

    % quaternion_to_dcm
    dcm00 = aSq + bSq - cSq - dSq;
    % dcm01 = 2*(b*c - a*d);
    dcm02 = 2*(a*c + b*d);
    dcm10 = 2*(b*c + a*d);
    % dcm11 = aSq - bSq + cSq - dSq;
    dcm12 = 2*(c*d - a*b);
    dcm20 = 2*(b*d - a*c);
    dcm21 = 2*(a*b + c*d);
    dcm22 = aSq - bSq - cSq + dSq;

    % dcm_to_euler
    theta = asin(-dcm20);
    if abs(theta - d_pi2) < 1.0e-3
        phi = single(0.0);
        psi = atan2(dcm12, dcm02);
    elseif abs(theta + d_pi2) < 1.0e-3
        phi = single(0.0);
        psi = atan2(-dcm12, -dcm02);
    else
        phi = atan2(dcm21, dcm22);
        psi = atan2(dcm10, dcm00);
    end

end

== matlab function AttitudeControl_ADRC_FLY/Control System1/pwm_out2 ==
  data: Roll input; M1 output; Pitch input; Yaw input; Thrust input; M2 output; M3 output; M4 output
function [M1, M2, M3, M4] = motor_mixer(Roll, Pitch, Yaw, Thrust)
%Function description:
%  Control allocation. The quadrotor type is X-configuration,
%  and the airframe is as follows:
%3↓   1↑
 %  \ /
 %  / \
 %2↑   4↓
%Input：
%  Roll, Pitch, Yaw: attitude controller output.
%  Thrust

idle_PWM = 0;
scale = 1;

M1 = (Thrust - Roll + Pitch + Yaw) * scale + idle_PWM;
M2 = (Thrust + Roll - Pitch + Yaw) * scale + idle_PWM;
M3 = (Thrust + Roll + Pitch - Yaw) * scale + idle_PWM;
M4 = (Thrust - Roll - Pitch - Yaw) * scale + idle_PWM;
if M1 < 0
    M1 = single(0);
elseif M1 > 1
    M1 = single(1);  
end
if M2 < 0
    M2 = single(0);
elseif M2 > 1
    M2 = single(1);  
end
if M3<0
    M3 = single(0);
elseif M3 > 1
    M3 = single(1);  
end
if M4<0
    M4 = single(0);
elseif M4 > 1
    M4 = single(1);  
end

== matlab function AttitudeControl_ADRC_FLY/Control System1/AttitudeControl/TD/get_dt ==
  data: timestamp input; dt output
function dt = get_dt(timestamp)
%timestamp: s
%dt :s
persistent t_last
if isempty(t_last)
    t_last = timestamp;
end
dt = timestamp - t_last;
t_last = timestamp;

== matlab function AttitudeControl_ADRC_FLY/Control System1/AttitudeControl/NLSEF/fhan ==
  data: x1 input single; y output single; x2 input single; r input single; h input single
function y = fhan(x1, x2, r, h)
    d = r * h^2;
    a0 = h * x2;
    y = x1 + a0;
    a1 = sqrt( d * (d + 8*abs(y)) );
    a2 = a0 + sign(y)*(a1 - d)/2;
    sy = (sign(y + d) - sign(y - d))/2;
    a = (a0 + y - a2)*sy + a2;
    sa = (sign(a + d) - sign(a - d))/2;
    y = -r*(a/d - sign(a))*sa - r*sign(a);

== matlab function AttitudeControl_ADRC_FLY/Control System1/AttitudeControl/TD/TD ==
  data: v input; v1_ output; r input; h input; v2_ output
function [v1_, v2_] = TD(v, r, h)
persistent v1 v2
if isempty(v1) || isempty(v2)
    v1 = 0;
    v2 = 0;
end

fv = fhan(v1 - v, v2, r,  h);
v1_ = v1 + h*v2;
v2_ = v2 + h*fv;

v1 = v1_;
v2 = v2_;
end

function y = fhan(x1, x2, r0, h0)

d = r0*h0^2;
a0 = h0*x2;
y = x1 + a0;
a1 = sqrt(d*(d + 8*abs(y)));
a2 = a0 + sign(y)*(a1 - d)/2;
sy = (sign(y + d) - sign(y - d))/2;%fsg
a = (a0 + y -a2)*sy + a2;
sa = (sign(a + d) - sign(a - d))/2;
y = -r0*(a/d - sign(a))*sa - r0*sign(a);

end

== matlab function AttitudeControl_ADRC_FLY/Control System1/AttitudeControl/ESO/adrc_eso ==
  data: y input; u input; z1_ output; b01 input; b02 input; b03 input; b0 input; d input; h input; z2_ output; z3_ output
function [z1_, z2_, z3_] = adrc_eso(y, u, b01, b02, b03, b0, d, h)
persistent z1  z2 z3
if (isempty(z1) || isempty(z2) || isempty(z3))
    z1 = 0;
    z2 = 0;
    z3 = 0;
end
e = z1 - y;
fe = fal(e, 0.5, d);
fe1 = fal(e, 0.25, d);

z1_ = z1 + h*(z2 - b01*e);
z2_ = z2 + h*(z3 + b0*u - b02*fe);
z3_ = z3 - h*b03*fe1;

z1 = z1_;
z2 = z2_;
z3 = z3_;

end

function  y = fal( x, alpha, delta )

if abs(x) < delta
    y = x / delta^(1.0 - alpha);
else
    y = (abs(x)^alpha) * sign(x);
end

end

== matlab function AttitudeControl_ADRC_FLY/Control System1/InputConditioning/f1 ==
  data: in input; y output; hover input
function y = thr_curve(in, hover)
%Function description:
%  After this function, when the throttle is in the middle position, the output is hovering throttle hover
%Input:
%  in: Throttle normalized value, range (0~1)
%  hover: Hovering throttle value
%Output:
%  Processed throttle value
if in < 0.5
	y=2 * in * hover;
else
	y=hover + 2 * (in - 0.5) * (1.0 - hover);
end
